simulink model "fig7_73"  (Simulink 4.00)
settings: Solver=ode23  StartTime=0.0  StopTime=300.0  RelTol=1e-6
settings Model: LastModifiedBy=abbas  LimitDataPoints=off  ExtModeTrigMode=oneshot  ExtModeArmWhenConnect=off  BlockReductionOpt=off

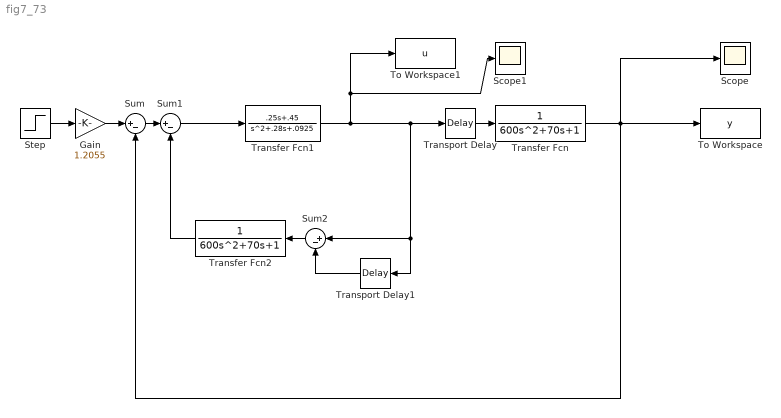
== system fig7_73 ==
  Gain : Gain  Gain=1.2055  Multiplication=Element-wise(K.*u)  SaturateOnIntegerOverflow=on
  Scope : Scope
      settings: TimeRange=auto  YMin=-5  YMax=5  SaveToWorkspace=off  SaveName=ScopeData  LimitDataPoints=on  MaxDataPoints=5000
  Scope1 : Scope
      settings: TimeRange=auto  YMin=-5  YMax=5  SaveToWorkspace=off  SaveName=ScopeData  LimitDataPoints=on  MaxDataPoints=5000
  Step : Step  Time=1  Before=0  After=1  SampleTime=0
  Sum : Sum  Inputs=|+-  SaturateOnIntegerOverflow=on
  Sum1 : Sum  Inputs=|+-  SaturateOnIntegerOverflow=on
  Sum2 : Sum  Orientation=left  Inputs=|+-  SaturateOnIntegerOverflow=on
  To Workspace : ToWorkspace  VariableName=y  SampleTime=-1  SaveFormat=Array
  To Workspace1 : ToWorkspace  VariableName=u  SampleTime=-1  SaveFormat=Array
  Transfer Fcn : TransferFcn  Numerator=[1]  Denominator=[600 70 1]  Realization=auto  AbsoluteTolerance=auto
  Transfer Fcn1 : TransferFcn  Numerator="[.25  .45]"  Denominator=[1 .28 .0925]  Realization=auto  AbsoluteTolerance=auto
  Transfer Fcn2 : TransferFcn  Orientation=left  Numerator=[1]  Denominator=[600 70 1]  Realization=auto  AbsoluteTolerance=auto
  Transport Delay : TransportDelay  DelayTime=5  InitialInput=0  BufferSize=1024  PadeOrder=0
  Transport Delay1 : TransportDelay  Orientation=left  DelayTime=5  InitialInput=0  BufferSize=1024  PadeOrder=0
  wires:
  Transport Delay/1 -> Transfer Fcn/1
  Transfer Fcn/1 -> To Workspace/1, Scope/1, Sum/2
  Sum1/1 -> Transfer Fcn1/1
  Sum/1 -> Sum1/1
  Transfer Fcn2/1 -> Sum1/2
  Sum2/1 -> Transfer Fcn2/1
  Transport Delay1/1 -> Sum2/2
  Transfer Fcn1/1 -> Transport Delay/1, Transport Delay1/1, Sum2/1, To Workspace1/1, Scope1/1
  Step/1 -> Gain/1
  Gain/1 -> Sum/1
